simulink library "tqd"  (R2021b)
settings: Solver=VariableStepAuto  StartTime=0.0  StopTime=10.0  RelTol=1e-3
undefined symbols (not defined in the file or in its folder): ATQD_AccelLimitInRange_X_rpm, ATQD_AccelLimitInRange_Y_Nm, ATQD_AccelLimitOvrKi_X_Nm, ATQD_AccelLimitOvrKp_X_Nm, ATQD_BOSMapD_X_rpm, ATQD_BOSMapD_Y_pct, ATQD_BOSMapR_X_rpm, ATQD_BOSMapR_Y_pct, ATQD_HVBCurrSmooth_X_A, ATQD_LHMTqMapDLC_X_rpm, ATQD_LHMTqMapDLC_Y_pct, ATQD_LHMTqMapRLC_X_rpm, ATQD_LHMTqMapRLC_Y_pct, ATQD_NormalMapDLC_X_rpm, ATQD_NormalMapDLC_Y_pct, ATQD_NormalTqDecSR_X_rpm, ATQD_NormalTqDecSR_Y_Nm, ATQD_NormalTqIncSR_X_rpm, ATQD_NormalTqIncSR_Y_Nm, ATQD_OPDMapRLC_X_rpm, ATQD_OPDMapRLC_Y_pct, ATQD_RollRegTorReq_X_rpm, ATQD_RollRegTorReq_Y_enum, ATQD_VehSpdLimitInRange_X_rpm, ATQD_VehSpdLimitInRange_Y_Nm, ATQD_VehSpdLimitOvrKi_X_Nm, ATQD_VehSpdLimitOvrKp_X_Nm, EIGHT_INT, ENUM_BRAKEPEDAL_PRESSED, ENUM_BRAKEPEDAL_RELEASED, ENUM_COMBOKEY_DOWN, ENUM_COMBOKEY_M1, ENUM_COMBOKEY_M2, ENUM_COMBOKEY_NONE, ENUM_COMBOKEY_RKNEE, ENUM_COMBOKEY_STOPLV, ENUM_COMBOKEY_UP, ENUM_CP2VKNEEREQ_REQUEST, ENUM_CP2VNLVREQ_LEVEL1, ENUM_CP2VNLVREQ_LEVEL2, ENUM_CP2VNLVREQ_LOWER, ENUM_CP2VNLVREQ_STOPLV, ENUM_CP2VNLVREQ_UPPER, ENUM_CREEPIND_DISABLE, ENUM_CREEPIND_READY, ENUM_CREEPIND_RUNNING, ENUM_CREEPIND_WARNING, ENUM_DRIVELINERELEASE_RELEASE, ENUM_EBSTORQUERWQ_LIMIT, ENUM_EBSTORQUERWQ_TORQUE, ENUM_ECPVCUDRM_CONFORT, ENUM_ECPVCUDRM_ECO, ENUM_ECPVCUDRM_NORMAL, ENUM_ECPVCUDRM_NOTAVAILABLE, ENUM_EMTqModeDrvBrk_Accel, ENUM_EMTqModeDrvBrk_Brake, ENUM_EMTqModeDrvBrk_Coast, ENUM_ETC2ACTDRIVEDIR_BACKWARD, ENUM_ETC2ACTDRIVEDIR_FORWARD, ENUM_ETC2ACTDRIVEDIR_STILL ... (+341)
libraries: simulink x109, hcu_lib x67
(part 12 of 13)

== system tqd/TQD/Input_Convert/Input Signal Convert/Big Mike Combo V2 /Combo Key Detection/Function5/Key4 ==
  VTQD_ComboKeyCMD_enum : Inport
  VTQD_ComboKeyEn_flg : Inport  Port=2
  VTQD_ComboKeyReset_flg : Inport  Port=3
  VTQD_ComboKey3_enum : Inport  Port=4
  AND : Logic  Inputs=4  AllPortsSameDT=off  OutDataTypeStr=boolean
  Constant1 : Constant  Value=KTQD_Function5Off4_enum
  Constant2 : Constant  Value=ENUM_COMBOKEY_NONE
  Constant3 : Constant  Value=ENUM_COMBOKEY_NONE
  Constant4 : Constant  Value=ENUM_COMBOKEY_NONE
  Data Type Conversion : DataTypeConversion  OutDataTypeStr=uint8
  Delay : Delay  DelayLength=1  InitialCondition=uint8(0)
      settings: AttributesFormatString=%<InitialCondition>
  Delay1 : Delay  DelayLength=1  InitialCondition=uint8(0)
      settings: AttributesFormatString=%<InitialCondition>
  Delay2 : Delay  DelayLength=1  InitialCondition=uint8(0)
      settings: AttributesFormatString=%<InitialCondition>
  Detect Change : simulink/Logic and Bit Operations/Detect Change  vinit=boolean(0)  OutDataTypeStr=boolean
  Detect Increase : simulink/Logic and Bit Operations/Detect Increase  vinit=boolean(0)  OutDataTypeStr=boolean
  Equal : RelationalOperator  Operator===  OutDataTypeStr=boolean  RndMeth=Simplest
  Equal1 : RelationalOperator  Operator=~=  OutDataTypeStr=boolean  RndMeth=Simplest
  Equal2 : RelationalOperator  Operator=~=  OutDataTypeStr=boolean  RndMeth=Simplest
  Equal3 : RelationalOperator  Operator===  OutDataTypeStr=boolean  RndMeth=Simplest
  If : If  NumInputs=2  IfExpression=u1 ~=0  ElseIfExpressions=u2 ~= 0
  Maintain : Subsystem  TreatAsAtomicUnit=on
  Merge : Merge  Inputs=3
  OR : Logic  Operator=OR  AllPortsSameDT=off  OutDataTypeStr=boolean
  Reset : Subsystem  TreatAsAtomicUnit=on
  Write : Subsystem  TreatAsAtomicUnit=on
  VTQD_ComboKey4_enum : Outport
  VTQD_Key4Pass_flg : Outport  Port=2
  wires:
  [VTQD_ComboKey4_enum] -> Equal/1
  VTQD_ComboKeyEn_flg/1 -> [VTQD_ComboKeyEn_flg]
  VTQD_ComboKeyReset_flg/1 -> [VTQD_ComboKeyReset_flg]
  VTQD_ComboKeyCMD_enum/1 -> [VTQD_ComboKeyCMD_enum]
  Equal/1 -> [VTQD_Key4Pass_flg]  "VTQD_Function5Off4Pass_flg"
  Constant1/1 -> Equal/2
  If/2 -> Write/Action
  Write/1(WriteCMD) -> Merge/2
  If/1 -> Reset/Action
  Detect Increase/1 -> OR/1
  AND/1 -> [VTQD_WriteComboCMD_flg]  "VTQD_WriteComboCMD_flg"
  [VTQD_ComboKeyCMD_enum] -> Write/1(Input)
  [VTQD_ComboKeyCMD_enum] -> Detect Change/1
  [VTQD_ResetComboKey_flg] -> If/1
  [VTQD_ComboKeyEn_flg] -> Detect Increase/1
  Detect Change/1 -> AND/1
  Maintain/1(KeepKey4) -> Merge/3
  Constant4/1 -> Equal1/2
  If/3 -> Maintain/Action
  Delay/1 -> Equal2/1
  Merge/1 -> Data Type Conversion/1
  Reset/1(ResetToZero) -> Merge/1
  Equal2/1 -> AND/3
  Constant2/1 -> Equal2/2
  Equal1/1 -> AND/2
  [VTQD_ComboKey3_enum] -> Delay/1
  [VTQD_ComboKeyReset_flg] -> OR/2
  [VTQD_ComboKeyCMD_enum] -> Equal1/1
  [VTQD_WriteComboCMD_flg] -> If/2
  OR/1 -> [VTQD_ResetComboKey_flg]  "VTQD_ResetComboKey_flg"
  VTQD_ComboKey3_enum/1 -> [VTQD_ComboKey3_enum]
  [VTQD_ComboKey4_enum] -> Delay1/1
  Constant3/1 -> Equal3/2
  Delay1/1 -> Equal3/1
  Equal3/1 -> AND/4
  [VTQD_Key4Pass_flg] -> VTQD_Key4Pass_flg/1
  [VTQD_ComboKey4_enum] -> VTQD_ComboKey4_enum/1
  [VTQD_ComboKey4_enum] -> Delay2/1
  Delay2/1 -> Maintain/1(Input)
  Data Type Conversion/1 -> [VTQD_ComboKey4_enum]  "VTQD_Function5Off4_enum"

== system tqd/TQD/Input_Convert/Input Signal Convert/Big Mike Combo V2 /Combo Key Detection/Function5/Key5 ==
  VTQD_ComboKeyCMD_enum : Inport
  VTQD_ComboKeyEn_flg : Inport  Port=2
  VTQD_ComboKeyReset_flg : Inport  Port=3
  VTQD_ComboKey4_enum : Inport  Port=4
  AND : Logic  Inputs=4  AllPortsSameDT=off  OutDataTypeStr=boolean
  Constant1 : Constant  Value=KTQD_Function5Off5_enum
  Constant2 : Constant  Value=ENUM_COMBOKEY_NONE
  Constant3 : Constant  Value=ENUM_COMBOKEY_NONE
  Constant4 : Constant  Value=ENUM_COMBOKEY_NONE
  Data Type Conversion : DataTypeConversion  OutDataTypeStr=uint8
  Delay : Delay  DelayLength=1  InitialCondition=uint8(0)
      settings: AttributesFormatString=%<InitialCondition>
  Delay1 : Delay  DelayLength=1  InitialCondition=uint8(0)
      settings: AttributesFormatString=%<InitialCondition>
  Delay2 : Delay  DelayLength=1  InitialCondition=uint8(0)
      settings: AttributesFormatString=%<InitialCondition>
  Detect Change : simulink/Logic and Bit Operations/Detect Change  vinit=boolean(0)  OutDataTypeStr=boolean
  Detect Increase : simulink/Logic and Bit Operations/Detect Increase  vinit=boolean(0)  OutDataTypeStr=boolean
  Equal : RelationalOperator  Operator===  OutDataTypeStr=boolean  RndMeth=Simplest
  Equal1 : RelationalOperator  Operator=~=  OutDataTypeStr=boolean  RndMeth=Simplest
  Equal2 : RelationalOperator  Operator=~=  OutDataTypeStr=boolean  RndMeth=Simplest
  Equal3 : RelationalOperator  Operator===  OutDataTypeStr=boolean  RndMeth=Simplest
  If : If  NumInputs=2  IfExpression=u1 ~=0  ElseIfExpressions=u2 ~= 0
  Maintain : Subsystem  TreatAsAtomicUnit=on
  Merge : Merge  Inputs=3
  OR : Logic  Operator=OR  AllPortsSameDT=off  OutDataTypeStr=boolean
  Reset : Subsystem  TreatAsAtomicUnit=on
  Write : Subsystem  TreatAsAtomicUnit=on
  VTQD_ComboKey5_enum : Outport
  VTQD_Key5Pass_flg : Outport  Port=2
  wires:
  [VTQD_Key5Pass_flg] -> VTQD_Key5Pass_flg/1
  Equal3/1 -> AND/4
  Delay1/1 -> Equal3/1
  Constant3/1 -> Equal3/2
  [VTQD_ComboKey5_enum] -> Delay1/1
  VTQD_ComboKey4_enum/1 -> [VTQD_ComboKey4_enum]
  OR/1 -> [VTQD_ResetComboKey_flg]  "VTQD_ResetComboKey_flg"
  [VTQD_WriteComboCMD_flg] -> If/2
  [VTQD_ComboKeyCMD_enum] -> Equal1/1
  [VTQD_ComboKeyReset_flg] -> OR/2
  [VTQD_ComboKey4_enum] -> Delay/1
  Equal1/1 -> AND/2
  Constant2/1 -> Equal2/2
  Equal2/1 -> AND/3
  Reset/1(ResetToZero) -> Merge/1
  Merge/1 -> Data Type Conversion/1
  Delay/1 -> Equal2/1
  If/3 -> Maintain/Action
  Constant4/1 -> Equal1/2
  Maintain/1(KeepKey5) -> Merge/3
  Detect Change/1 -> AND/1
  [VTQD_ComboKeyEn_flg] -> Detect Increase/1
  [VTQD_ResetComboKey_flg] -> If/1
  [VTQD_ComboKeyCMD_enum] -> Detect Change/1
  [VTQD_ComboKeyCMD_enum] -> Write/1(Input)
  AND/1 -> [VTQD_WriteComboCMD_flg]  "VTQD_WriteComboCMD_flg"
  Detect Increase/1 -> OR/1
  If/1 -> Reset/Action
  Write/1(WriteCMD) -> Merge/2
  If/2 -> Write/Action
  Constant1/1 -> Equal/2
  Equal/1 -> [VTQD_Key5Pass_flg]  "VTQD_Function5Off5Pass_flg"
  VTQD_ComboKeyCMD_enum/1 -> [VTQD_ComboKeyCMD_enum]
  VTQD_ComboKeyReset_flg/1 -> [VTQD_ComboKeyReset_flg]
  VTQD_ComboKeyEn_flg/1 -> [VTQD_ComboKeyEn_flg]
  [VTQD_ComboKey5_enum] -> Equal/1
  [VTQD_ComboKey5_enum] -> VTQD_ComboKey5_enum/1
  [VTQD_ComboKey5_enum] -> Delay2/1
  Delay2/1 -> Maintain/1(Input)
  Data Type Conversion/1 -> [VTQD_ComboKey5_enum]  "VTQD_Function5Off5_enum"

== system tqd/TQD/Input_Convert/Input Signal Convert/Big Mike Combo V2 /Combo Key Detection/Function5/Key6 ==
  VTQD_ComboKeyCMD_enum : Inport
  VTQD_ComboKeyEn_flg : Inport  Port=2
  VTQD_ComboKeyReset_flg : Inport  Port=3
  VTQD_ComboKey5_enum : Inport  Port=4
  AND : Logic  Inputs=4  AllPortsSameDT=off  OutDataTypeStr=boolean
  Constant1 : Constant  Value=KTQD_Function5Off6_enum
  Constant2 : Constant  Value=ENUM_COMBOKEY_NONE
  Constant3 : Constant  Value=ENUM_COMBOKEY_NONE
  Constant4 : Constant  Value=ENUM_COMBOKEY_NONE
  Data Type Conversion : DataTypeConversion  OutDataTypeStr=uint8
  Delay : Delay  DelayLength=1  InitialCondition=uint8(0)
      settings: AttributesFormatString=%<InitialCondition>
  Delay1 : Delay  DelayLength=1  InitialCondition=uint8(0)
      settings: AttributesFormatString=%<InitialCondition>
  Delay2 : Delay  DelayLength=1  InitialCondition=uint8(0)
      settings: AttributesFormatString=%<InitialCondition>
  Detect Change : simulink/Logic and Bit Operations/Detect Change  vinit=boolean(0)  OutDataTypeStr=boolean
  Detect Increase : simulink/Logic and Bit Operations/Detect Increase  vinit=boolean(0)  OutDataTypeStr=boolean
  Equal : RelationalOperator  Operator===  OutDataTypeStr=boolean  RndMeth=Simplest
  Equal1 : RelationalOperator  Operator=~=  OutDataTypeStr=boolean  RndMeth=Simplest
  Equal2 : RelationalOperator  Operator=~=  OutDataTypeStr=boolean  RndMeth=Simplest
  Equal3 : RelationalOperator  Operator===  OutDataTypeStr=boolean  RndMeth=Simplest
  If : If  NumInputs=2  IfExpression=u1 ~=0  ElseIfExpressions=u2 ~= 0
  Maintain : Subsystem  TreatAsAtomicUnit=on
  Merge : Merge  Inputs=3
  OR : Logic  Operator=OR  AllPortsSameDT=off  OutDataTypeStr=boolean
  Reset : Subsystem  TreatAsAtomicUnit=on
  Write : Subsystem  TreatAsAtomicUnit=on
  VTQD_ComboKey6_enum : Outport
  VTQD_Key6Pass_flg : Outport  Port=2
  wires:
  [VTQD_ComboKey6_enum] -> VTQD_ComboKey6_enum/1
  [VTQD_ComboKey6_enum] -> Equal/1
  VTQD_ComboKeyEn_flg/1 -> [VTQD_ComboKeyEn_flg]
  VTQD_ComboKeyReset_flg/1 -> [VTQD_ComboKeyReset_flg]
  VTQD_ComboKeyCMD_enum/1 -> [VTQD_ComboKeyCMD_enum]
  Equal/1 -> [VTQD_Key6Pass_flg]  "VTQD_Function5Off6Pass_flg"
  Constant1/1 -> Equal/2
  If/2 -> Write/Action
  Write/1(WriteCMD) -> Merge/2
  If/1 -> Reset/Action
  Detect Increase/1 -> OR/1
  AND/1 -> [VTQD_WriteComboCMD_flg]  "VTQD_WriteComboCMD_flg"
  [VTQD_ComboKeyCMD_enum] -> Write/1(Input)
  [VTQD_ComboKeyCMD_enum] -> Detect Change/1
  [VTQD_ResetComboKey_flg] -> If/1
  [VTQD_ComboKeyEn_flg] -> Detect Increase/1
  Detect Change/1 -> AND/1
  Maintain/1(KeepKey6) -> Merge/3
  Constant4/1 -> Equal1/2
  If/3 -> Maintain/Action
  Delay/1 -> Equal2/1
  Merge/1 -> Data Type Conversion/1
  Reset/1(ResetToZero) -> Merge/1
  Equal2/1 -> AND/3
  Constant2/1 -> Equal2/2
  Equal1/1 -> AND/2
  [VTQD_ComboKey5_enum] -> Delay/1
  [VTQD_ComboKeyReset_flg] -> OR/2
  [VTQD_ComboKeyCMD_enum] -> Equal1/1
  [VTQD_WriteComboCMD_flg] -> If/2
  OR/1 -> [VTQD_ResetComboKey_flg]  "VTQD_ResetComboKey_flg"
  VTQD_ComboKey5_enum/1 -> [VTQD_ComboKey5_enum]
  [VTQD_ComboKey6_enum] -> Delay1/1
  Constant3/1 -> Equal3/2
  Delay1/1 -> Equal3/1
  Equal3/1 -> AND/4
  [VTQD_Key6Pass_flg] -> VTQD_Key6Pass_flg/1
  Delay2/1 -> Maintain/1(Input)
  [VTQD_ComboKey6_enum] -> Delay2/1
  Data Type Conversion/1 -> [VTQD_ComboKey6_enum]  "VTQD_Function5Off6_enum"

== system tqd/TQD/Input_Convert/Input Signal Convert/Big Mike Combo V2 /Combo Key Detection/Function5/Key7 ==
  VTQD_ComboKeyCMD_enum : Inport
  VTQD_ComboKeyEn_flg : Inport  Port=2
  VTQD_ComboKeyReset_flg : Inport  Port=3
  VTQD_ComboKey6_enum : Inport  Port=4
  AND : Logic  Inputs=4  AllPortsSameDT=off  OutDataTypeStr=boolean
  Constant1 : Constant  Value=KTQD_Function5Off7_enum
  Constant2 : Constant  Value=ENUM_COMBOKEY_NONE  OutDataTypeStr=uint8
  Constant3 : Constant  Value=ENUM_COMBOKEY_NONE
  Constant4 : Constant  Value=ENUM_COMBOKEY_NONE  OutDataTypeStr=uint8
  Data Type Conversion : DataTypeConversion  OutDataTypeStr=uint8
  Delay : Delay  DelayLength=1  InitialCondition=uint8(0)
      settings: AttributesFormatString=%<InitialCondition>
  Delay1 : Delay  DelayLength=1  InitialCondition=uint8(0)
      settings: AttributesFormatString=%<InitialCondition>
  Delay2 : Delay  DelayLength=1  InitialCondition=uint8(0)
      settings: AttributesFormatString=%<InitialCondition>
  Detect Change : simulink/Logic and Bit Operations/Detect Change  vinit=boolean(0)  OutDataTypeStr=boolean
  Detect Increase : simulink/Logic and Bit Operations/Detect Increase  vinit=boolean(0)  OutDataTypeStr=boolean
  Equal : RelationalOperator  Operator===  OutDataTypeStr=boolean  RndMeth=Simplest
  Equal1 : RelationalOperator  Operator=~=  OutDataTypeStr=boolean  RndMeth=Simplest
  Equal2 : RelationalOperator  Operator=~=  OutDataTypeStr=boolean  RndMeth=Simplest
  Equal3 : RelationalOperator  Operator===  OutDataTypeStr=boolean  RndMeth=Simplest
  If : If  NumInputs=2  IfExpression=u1 ~=0  ElseIfExpressions=u2 ~= 0
  Maintain : Subsystem  TreatAsAtomicUnit=on
  Merge : Merge  Inputs=3
  OR : Logic  Operator=OR  AllPortsSameDT=off  OutDataTypeStr=boolean
  Reset : Subsystem  TreatAsAtomicUnit=on
  Write : Subsystem  TreatAsAtomicUnit=on
  VTQD_ComboKey7_enum : Outport
  VTQD_Key7Pass_flg : Outport  Port=2
  wires:
  [VTQD_Key7Pass_flg] -> VTQD_Key7Pass_flg/1
  Equal3/1 -> AND/4
  Delay1/1 -> Equal3/1
  Constant3/1 -> Equal3/2
  [VTQD_ComboKey7_enum] -> Delay1/1
  VTQD_ComboKey6_enum/1 -> [VTQD_ComboKey6_enum]
  OR/1 -> [VTQD_ResetComboKey_flg]  "VTQD_ResetComboKey_flg"
  [VTQD_WriteComboCMD_flg] -> If/2
  [VTQD_ComboKeyCMD_enum] -> Equal1/1
  [VTQD_ComboKeyReset_flg] -> OR/2
  [VTQD_ComboKey6_enum] -> Delay/1
  Equal1/1 -> AND/2
  Constant2/1 -> Equal2/2
  Equal2/1 -> AND/3
  Reset/1(ResetToZero) -> Merge/1
  Merge/1 -> Data Type Conversion/1
  Delay/1 -> Equal2/1
  If/3 -> Maintain/Action
  Constant4/1 -> Equal1/2
  Maintain/1(KeepKey7) -> Merge/3
  Detect Change/1 -> AND/1
  [VTQD_ComboKeyEn_flg] -> Detect Increase/1
  [VTQD_ResetComboKey_flg] -> If/1
  [VTQD_ComboKeyCMD_enum] -> Detect Change/1
  [VTQD_ComboKeyCMD_enum] -> Write/1(Input)
  AND/1 -> [VTQD_WriteComboCMD_flg]  "VTQD_WriteComboCMD_flg"
  Detect Increase/1 -> OR/1
  If/1 -> Reset/Action
  Write/1(WriteCMD) -> Merge/2
  If/2 -> Write/Action
  Constant1/1 -> Equal/2
  Equal/1 -> [VTQD_Key7Pass_flg]  "VTQD_Function5Off7Pass_flg"
  VTQD_ComboKeyCMD_enum/1 -> [VTQD_ComboKeyCMD_enum]
  VTQD_ComboKeyReset_flg/1 -> [VTQD_ComboKeyReset_flg]
  VTQD_ComboKeyEn_flg/1 -> [VTQD_ComboKeyEn_flg]
  [VTQD_ComboKey7_enum] -> Equal/1
  [VTQD_ComboKey7_enum] -> VTQD_ComboKey7_enum/1
  [VTQD_ComboKey7_enum] -> Delay2/1
  Delay2/1 -> Maintain/1(Input)
  Data Type Conversion/1 -> [VTQD_ComboKey7_enum]  "VTQD_Function5Off7_enum"

== system tqd/TQD/Input_Convert/Input Signal Convert/Big Mike Combo V2 /Combo Key Detection/Function5/Key8 ==
  VTQD_ComboKeyCMD_enum : Inport
  VTQD_ComboKeyEn_flg : Inport  Port=2
  VTQD_ComboKeyReset_flg : Inport  Port=3
  VTQD_ComboKey7_enum : Inport  Port=4
  AND : Logic  Inputs=4  AllPortsSameDT=off  OutDataTypeStr=boolean
  Constant1 : Constant  Value=KTQD_Function5Off8_enum
  Constant2 : Constant  Value=ENUM_COMBOKEY_NONE
  Constant3 : Constant  Value=ENUM_COMBOKEY_NONE
  Constant4 : Constant  Value=ENUM_COMBOKEY_NONE
  Data Type Conversion : DataTypeConversion  OutDataTypeStr=uint8
  Delay : Delay  DelayLength=1  InitialCondition=uint8(0)
      settings: AttributesFormatString=%<InitialCondition>
  Delay1 : Delay  DelayLength=1  InitialCondition=uint8(0)
      settings: AttributesFormatString=%<InitialCondition>
  Delay2 : Delay  DelayLength=1  InitialCondition=uint8(0)
      settings: AttributesFormatString=%<InitialCondition>
  Detect Change : simulink/Logic and Bit Operations/Detect Change  vinit=boolean(0)  OutDataTypeStr=boolean
  Detect Increase : simulink/Logic and Bit Operations/Detect Increase  vinit=boolean(0)  OutDataTypeStr=boolean
  Equal : RelationalOperator  Operator===  OutDataTypeStr=boolean  RndMeth=Simplest
  Equal1 : RelationalOperator  Operator=~=  OutDataTypeStr=boolean  RndMeth=Simplest
  Equal2 : RelationalOperator  Operator=~=  OutDataTypeStr=boolean  RndMeth=Simplest
  Equal3 : RelationalOperator  Operator===  OutDataTypeStr=boolean  RndMeth=Simplest
  If : If  NumInputs=2  IfExpression=u1 ~=0  ElseIfExpressions=u2 ~= 0
  Maintain : Subsystem  TreatAsAtomicUnit=on
  Merge : Merge  Inputs=3
  OR : Logic  Operator=OR  AllPortsSameDT=off  OutDataTypeStr=boolean
  Reset : Subsystem  TreatAsAtomicUnit=on
  Write : Subsystem  TreatAsAtomicUnit=on
  VTQD_ComboKey8_enum : Outport
  VTQD_Key8Pass_flg : Outport  Port=2
  wires:
  VTQD_ComboKeyEn_flg/1 -> [VTQD_ComboKeyEn_flg]
  VTQD_ComboKeyReset_flg/1 -> [VTQD_ComboKeyReset_flg]
  VTQD_ComboKeyCMD_enum/1 -> [VTQD_ComboKeyCMD_enum]
  Equal/1 -> [VTQD_Key8Pass_flg]  "VTQD_Function5Off8Pass_flg"
  Constant1/1 -> Equal/2
  If/2 -> Write/Action
  Write/1(WriteCMD) -> Merge/2
  If/1 -> Reset/Action
  Detect Increase/1 -> OR/1
  AND/1 -> [VTQD_WriteComboCMD_flg]  "VTQD_WriteComboCMD_flg"
  [VTQD_ComboKeyCMD_enum] -> Write/1(Input)
  [VTQD_ComboKeyCMD_enum] -> Detect Change/1
  [VTQD_ResetComboKey_flg] -> If/1
  [VTQD_ComboKeyEn_flg] -> Detect Increase/1
  Detect Change/1 -> AND/1
  Maintain/1(KeepKey8) -> Merge/3
  Constant4/1 -> Equal1/2
  If/3 -> Maintain/Action
  Delay/1 -> Equal2/1
  Merge/1 -> Data Type Conversion/1
  Reset/1(ResetToZero) -> Merge/1
  Equal2/1 -> AND/3
  Constant2/1 -> Equal2/2
  Equal1/1 -> AND/2
  [VTQD_ComboKey7_enum] -> Delay/1
  [VTQD_ComboKeyReset_flg] -> OR/2
  [VTQD_ComboKeyCMD_enum] -> Equal1/1
  [VTQD_WriteComboCMD_flg] -> If/2
  OR/1 -> [VTQD_ResetComboKey_flg]  "VTQD_ResetComboKey_flg"
  VTQD_ComboKey7_enum/1 -> [VTQD_ComboKey7_enum]
  [VTQD_ComboKey8_enum] -> Delay1/1
  Constant3/1 -> Equal3/2
  Delay1/1 -> Equal3/1
  Equal3/1 -> AND/4
  [VTQD_Key8Pass_flg] -> VTQD_Key8Pass_flg/1
  [VTQD_ComboKey8_enum] -> Equal/1
  [VTQD_ComboKey8_enum] -> VTQD_ComboKey8_enum/1
  [VTQD_ComboKey8_enum] -> Delay2/1
  Delay2/1 -> Maintain/1(Input)
  Data Type Conversion/1 -> [VTQD_ComboKey8_enum]  "VTQD_Function5Off8_enum"

== system tqd/TQD/Input_Convert/Input Signal Convert/Big Mike Combo V2 /Combo Key Detection/Function1 Alcohol Lock/Key1/Maintain ==
  Input : Inport
  Action Port : ActionPort
  KeepKey1 : Outport
  wires:
  Input/1 -> KeepKey1/1

== system tqd/TQD/Input_Convert/Input Signal Convert/Big Mike Combo V2 /Combo Key Detection/Function1 Alcohol Lock/Key1/Reset ==
  Action Port : ActionPort
  Constant : Constant  Value=ENUM_COMBOKEY_NONE
  ResetToZero : Outport
  wires:
  Constant/1 -> ResetToZero/1

== system tqd/TQD/Input_Convert/Input Signal Convert/Big Mike Combo V2 /Combo Key Detection/Function1 Alcohol Lock/Key1/Write ==
  Input : Inport
  Action Port : ActionPort
  WriteCMD : Outport
  wires:
  Input/1 -> WriteCMD/1

== system tqd/TQD/Input_Convert/Input Signal Convert/Big Mike Combo V2 /Combo Key Detection/Function1 Alcohol Lock/Key2/Maintain ==
  Input : Inport
  Action Port : ActionPort
  KeepKey2 : Outport
  wires:
  Input/1 -> KeepKey2/1

== system tqd/TQD/Input_Convert/Input Signal Convert/Big Mike Combo V2 /Combo Key Detection/Function1 Alcohol Lock/Key2/Reset ==
  Action Port : ActionPort
  Constant : Constant  Value=ENUM_COMBOKEY_NONE
  ResetToZero : Outport
  wires:
  Constant/1 -> ResetToZero/1

== system tqd/TQD/Input_Convert/Input Signal Convert/Big Mike Combo V2 /Combo Key Detection/Function1 Alcohol Lock/Key2/Write ==
  Input : Inport
  Action Port : ActionPort
  WriteCMD : Outport
  wires:
  Input/1 -> WriteCMD/1

== system tqd/TQD/Input_Convert/Input Signal Convert/Big Mike Combo V2 /Combo Key Detection/Function1 Alcohol Lock/Key3/Maintain ==
  Input : Inport
  Action Port : ActionPort
  KeepKey3 : Outport
  wires:
  Input/1 -> KeepKey3/1

== system tqd/TQD/Input_Convert/Input Signal Convert/Big Mike Combo V2 /Combo Key Detection/Function1 Alcohol Lock/Key3/Reset ==
  Action Port : ActionPort
  Constant : Constant  Value=ENUM_COMBOKEY_NONE
  ResetToZero : Outport
  wires:
  Constant/1 -> ResetToZero/1

== system tqd/TQD/Input_Convert/Input Signal Convert/Big Mike Combo V2 /Combo Key Detection/Function1 Alcohol Lock/Key3/Write ==
  Input : Inport
  Action Port : ActionPort
  WriteCMD : Outport
  wires:
  Input/1 -> WriteCMD/1

== system tqd/TQD/Input_Convert/Input Signal Convert/Big Mike Combo V2 /Combo Key Detection/Function1 Alcohol Lock/Key4/Maintain ==
  Input : Inport
  Action Port : ActionPort
  KeepKey4 : Outport
  wires:
  Input/1 -> KeepKey4/1

== system tqd/TQD/Input_Convert/Input Signal Convert/Big Mike Combo V2 /Combo Key Detection/Function1 Alcohol Lock/Key4/Reset ==
  Action Port : ActionPort
  Constant : Constant  Value=ENUM_COMBOKEY_NONE
  ResetToZero : Outport
  wires:
  Constant/1 -> ResetToZero/1

== system tqd/TQD/Input_Convert/Input Signal Convert/Big Mike Combo V2 /Combo Key Detection/Function1 Alcohol Lock/Key4/Write ==
  Input : Inport
  Action Port : ActionPort
  WriteCMD : Outport
  wires:
  Input/1 -> WriteCMD/1

== system tqd/TQD/Input_Convert/Input Signal Convert/Big Mike Combo V2 /Combo Key Detection/Function1 Alcohol Lock/Key5/Maintain ==
  Input : Inport
  Action Port : ActionPort
  KeepKey5 : Outport
  wires:
  Input/1 -> KeepKey5/1

== system tqd/TQD/Input_Convert/Input Signal Convert/Big Mike Combo V2 /Combo Key Detection/Function1 Alcohol Lock/Key5/Reset ==
  Action Port : ActionPort
  Constant : Constant  Value=ENUM_COMBOKEY_NONE
  ResetToZero : Outport
  wires:
  Constant/1 -> ResetToZero/1

== system tqd/TQD/Input_Convert/Input Signal Convert/Big Mike Combo V2 /Combo Key Detection/Function1 Alcohol Lock/Key5/Write ==
  Input : Inport
  Action Port : ActionPort
  WriteCMD : Outport
  wires:
  Input/1 -> WriteCMD/1

== system tqd/TQD/Input_Convert/Input Signal Convert/Big Mike Combo V2 /Combo Key Detection/Function1 Alcohol Lock/Key6/Maintain ==
  Input : Inport
  Action Port : ActionPort
  KeepKey6 : Outport
  wires:
  Input/1 -> KeepKey6/1

== system tqd/TQD/Input_Convert/Input Signal Convert/Big Mike Combo V2 /Combo Key Detection/Function1 Alcohol Lock/Key6/Reset ==
  Action Port : ActionPort
  Constant : Constant  Value=ENUM_COMBOKEY_NONE
  ResetToZero : Outport
  wires:
  Constant/1 -> ResetToZero/1

== system tqd/TQD/Input_Convert/Input Signal Convert/Big Mike Combo V2 /Combo Key Detection/Function1 Alcohol Lock/Key6/Write ==
  Input : Inport
  Action Port : ActionPort
  WriteCMD : Outport
  wires:
  Input/1 -> WriteCMD/1

== system tqd/TQD/Input_Convert/Input Signal Convert/Big Mike Combo V2 /Combo Key Detection/Function1 Alcohol Lock/Key7/Maintain ==
  Input : Inport
  Action Port : ActionPort
  KeepKey7 : Outport
  wires:
  Input/1 -> KeepKey7/1

== system tqd/TQD/Input_Convert/Input Signal Convert/Big Mike Combo V2 /Combo Key Detection/Function1 Alcohol Lock/Key7/Reset ==
  Action Port : ActionPort
  Constant : Constant  Value=ENUM_COMBOKEY_NONE
  ResetToZero : Outport
  wires:
  Constant/1 -> ResetToZero/1

== system tqd/TQD/Input_Convert/Input Signal Convert/Big Mike Combo V2 /Combo Key Detection/Function1 Alcohol Lock/Key7/Write ==
  Input : Inport
  Action Port : ActionPort
  WriteCMD : Outport
  wires:
  Input/1 -> WriteCMD/1

== system tqd/TQD/Input_Convert/Input Signal Convert/Big Mike Combo V2 /Combo Key Detection/Function1 Alcohol Lock/Key8/Maintain ==
  Input : Inport
  Action Port : ActionPort
  KeepKey8 : Outport
  wires:
  Input/1 -> KeepKey8/1

== system tqd/TQD/Input_Convert/Input Signal Convert/Big Mike Combo V2 /Combo Key Detection/Function1 Alcohol Lock/Key8/Reset ==
  Action Port : ActionPort
  Constant : Constant  Value=ENUM_COMBOKEY_NONE
  ResetToZero : Outport
  wires:
  Constant/1 -> ResetToZero/1

== system tqd/TQD/Input_Convert/Input Signal Convert/Big Mike Combo V2 /Combo Key Detection/Function1 Alcohol Lock/Key8/Write ==
  Input : Inport
  Action Port : ActionPort
  WriteCMD : Outport
  wires:
  Input/1 -> WriteCMD/1

== system tqd/TQD/Input_Convert/Input Signal Convert/Big Mike Combo V2 /Combo Key Detection/Function2 /Key1/Maintain ==
  Input : Inport
  Action Port : ActionPort
  KeepKey1 : Outport
  wires:
  Input/1 -> KeepKey1/1

== system tqd/TQD/Input_Convert/Input Signal Convert/Big Mike Combo V2 /Combo Key Detection/Function2 /Key1/Reset ==
  Action Port : ActionPort
  Constant : Constant  Value=ENUM_COMBOKEY_NONE
  ResetToZero : Outport
  wires:
  Constant/1 -> ResetToZero/1

== system tqd/TQD/Input_Convert/Input Signal Convert/Big Mike Combo V2 /Combo Key Detection/Function2 /Key1/Write ==
  Input : Inport
  Action Port : ActionPort
  WriteCMD : Outport
  wires:
  Input/1 -> WriteCMD/1

== system tqd/TQD/Input_Convert/Input Signal Convert/Big Mike Combo V2 /Combo Key Detection/Function2 /Key2/Maintain ==
  Input : Inport
  Action Port : ActionPort
  KeepKey2 : Outport
  wires:
  Input/1 -> KeepKey2/1

== system tqd/TQD/Input_Convert/Input Signal Convert/Big Mike Combo V2 /Combo Key Detection/Function2 /Key2/Reset ==
  Action Port : ActionPort
  Constant : Constant  Value=ENUM_COMBOKEY_NONE
  ResetToZero : Outport
  wires:
  Constant/1 -> ResetToZero/1

== system tqd/TQD/Input_Convert/Input Signal Convert/Big Mike Combo V2 /Combo Key Detection/Function2 /Key2/Write ==
  Input : Inport
  Action Port : ActionPort
  WriteCMD : Outport
  wires:
  Input/1 -> WriteCMD/1

== system tqd/TQD/Input_Convert/Input Signal Convert/Big Mike Combo V2 /Combo Key Detection/Function2 /Key3/Maintain ==
  Input : Inport
  Action Port : ActionPort
  KeepKey3 : Outport
  wires:
  Input/1 -> KeepKey3/1

== system tqd/TQD/Input_Convert/Input Signal Convert/Big Mike Combo V2 /Combo Key Detection/Function2 /Key3/Reset ==
  Action Port : ActionPort
  Constant : Constant  Value=ENUM_COMBOKEY_NONE
  ResetToZero : Outport
  wires:
  Constant/1 -> ResetToZero/1

== system tqd/TQD/Input_Convert/Input Signal Convert/Big Mike Combo V2 /Combo Key Detection/Function2 /Key3/Write ==
  Input : Inport
  Action Port : ActionPort
  WriteCMD : Outport
  wires:
  Input/1 -> WriteCMD/1

== system tqd/TQD/Input_Convert/Input Signal Convert/Big Mike Combo V2 /Combo Key Detection/Function2 /Key4/Maintain ==
  Input : Inport
  Action Port : ActionPort
  KeepKey4 : Outport
  wires:
  Input/1 -> KeepKey4/1

== system tqd/TQD/Input_Convert/Input Signal Convert/Big Mike Combo V2 /Combo Key Detection/Function2 /Key4/Reset ==
  Action Port : ActionPort
  Constant : Constant  Value=ENUM_COMBOKEY_NONE
  ResetToZero : Outport
  wires:
  Constant/1 -> ResetToZero/1

== system tqd/TQD/Input_Convert/Input Signal Convert/Big Mike Combo V2 /Combo Key Detection/Function2 /Key4/Write ==
  Input : Inport
  Action Port : ActionPort
  WriteCMD : Outport
  wires:
  Input/1 -> WriteCMD/1

== system tqd/TQD/Input_Convert/Input Signal Convert/Big Mike Combo V2 /Combo Key Detection/Function2 /Key5/Maintain ==
  Input : Inport
  Action Port : ActionPort
  KeepKey5 : Outport
  wires:
  Input/1 -> KeepKey5/1

== system tqd/TQD/Input_Convert/Input Signal Convert/Big Mike Combo V2 /Combo Key Detection/Function2 /Key5/Reset ==
  Action Port : ActionPort
  Constant : Constant  Value=ENUM_COMBOKEY_NONE
  ResetToZero : Outport
  wires:
  Constant/1 -> ResetToZero/1

== system tqd/TQD/Input_Convert/Input Signal Convert/Big Mike Combo V2 /Combo Key Detection/Function2 /Key5/Write ==
  Input : Inport
  Action Port : ActionPort
  WriteCMD : Outport
  wires:
  Input/1 -> WriteCMD/1

== system tqd/TQD/Input_Convert/Input Signal Convert/Big Mike Combo V2 /Combo Key Detection/Function2 /Key6/Maintain ==
  Input : Inport
  Action Port : ActionPort
  KeepKey6 : Outport
  wires:
  Input/1 -> KeepKey6/1

== system tqd/TQD/Input_Convert/Input Signal Convert/Big Mike Combo V2 /Combo Key Detection/Function2 /Key6/Reset ==
  Action Port : ActionPort
  Constant : Constant  Value=ENUM_COMBOKEY_NONE
  ResetToZero : Outport
  wires:
  Constant/1 -> ResetToZero/1

== system tqd/TQD/Input_Convert/Input Signal Convert/Big Mike Combo V2 /Combo Key Detection/Function2 /Key6/Write ==
  Input : Inport
  Action Port : ActionPort
  WriteCMD : Outport
  wires:
  Input/1 -> WriteCMD/1

== system tqd/TQD/Input_Convert/Input Signal Convert/Big Mike Combo V2 /Combo Key Detection/Function2 /Key7/Maintain ==
  Input : Inport
  Action Port : ActionPort
  KeepKey7 : Outport
  wires:
  Input/1 -> KeepKey7/1

== system tqd/TQD/Input_Convert/Input Signal Convert/Big Mike Combo V2 /Combo Key Detection/Function2 /Key7/Reset ==
  Action Port : ActionPort
  Constant : Constant  Value=ENUM_COMBOKEY_NONE
  ResetToZero : Outport
  wires:
  Constant/1 -> ResetToZero/1

== system tqd/TQD/Input_Convert/Input Signal Convert/Big Mike Combo V2 /Combo Key Detection/Function2 /Key7/Write ==
  Input : Inport
  Action Port : ActionPort
  WriteCMD : Outport
  wires:
  Input/1 -> WriteCMD/1

== system tqd/TQD/Input_Convert/Input Signal Convert/Big Mike Combo V2 /Combo Key Detection/Function2 /Key8/Maintain ==
  Input : Inport
  Action Port : ActionPort
  KeepKey8 : Outport
  wires:
  Input/1 -> KeepKey8/1

== system tqd/TQD/Input_Convert/Input Signal Convert/Big Mike Combo V2 /Combo Key Detection/Function2 /Key8/Reset ==
  Action Port : ActionPort
  Constant : Constant  Value=ENUM_COMBOKEY_NONE
  ResetToZero : Outport
  wires:
  Constant/1 -> ResetToZero/1

== system tqd/TQD/Input_Convert/Input Signal Convert/Big Mike Combo V2 /Combo Key Detection/Function2 /Key8/Write ==
  Input : Inport
  Action Port : ActionPort
  WriteCMD : Outport
  wires:
  Input/1 -> WriteCMD/1

== system tqd/TQD/Input_Convert/Input Signal Convert/Big Mike Combo V2 /Combo Key Detection/Function3/Key1/Maintain ==
  Input : Inport
  Action Port : ActionPort
  KeepKey1 : Outport
  wires:
  Input/1 -> KeepKey1/1

== system tqd/TQD/Input_Convert/Input Signal Convert/Big Mike Combo V2 /Combo Key Detection/Function3/Key1/Reset ==
  Action Port : ActionPort
  Constant : Constant  Value=ENUM_COMBOKEY_NONE
  ResetToZero : Outport
  wires:
  Constant/1 -> ResetToZero/1

== system tqd/TQD/Input_Convert/Input Signal Convert/Big Mike Combo V2 /Combo Key Detection/Function3/Key1/Write ==
  Input : Inport
  Action Port : ActionPort
  WriteCMD : Outport
  wires:
  Input/1 -> WriteCMD/1

== system tqd/TQD/Input_Convert/Input Signal Convert/Big Mike Combo V2 /Combo Key Detection/Function3/Key2/Maintain ==
  Input : Inport
  Action Port : ActionPort
  KeepKey2 : Outport
  wires:
  Input/1 -> KeepKey2/1

== system tqd/TQD/Input_Convert/Input Signal Convert/Big Mike Combo V2 /Combo Key Detection/Function3/Key2/Reset ==
  Action Port : ActionPort
  Constant : Constant  Value=ENUM_COMBOKEY_NONE
  ResetToZero : Outport
  wires:
  Constant/1 -> ResetToZero/1

== system tqd/TQD/Input_Convert/Input Signal Convert/Big Mike Combo V2 /Combo Key Detection/Function3/Key2/Write ==
  Input : Inport
  Action Port : ActionPort
  WriteCMD : Outport
  wires:
  Input/1 -> WriteCMD/1

== system tqd/TQD/Input_Convert/Input Signal Convert/Big Mike Combo V2 /Combo Key Detection/Function3/Key3/Maintain ==
  Input : Inport
  Action Port : ActionPort
  KeepKey3 : Outport
  wires:
  Input/1 -> KeepKey3/1

== system tqd/TQD/Input_Convert/Input Signal Convert/Big Mike Combo V2 /Combo Key Detection/Function3/Key3/Reset ==
  Action Port : ActionPort
  Constant : Constant  Value=ENUM_COMBOKEY_NONE
  ResetToZero : Outport
  wires:
  Constant/1 -> ResetToZero/1

== system tqd/TQD/Input_Convert/Input Signal Convert/Big Mike Combo V2 /Combo Key Detection/Function3/Key3/Write ==
  Input : Inport
  Action Port : ActionPort
  WriteCMD : Outport
  wires:
  Input/1 -> WriteCMD/1

== system tqd/TQD/Input_Convert/Input Signal Convert/Big Mike Combo V2 /Combo Key Detection/Function3/Key4/Maintain ==
  Input : Inport
  Action Port : ActionPort
  KeepKey4 : Outport
  wires:
  Input/1 -> KeepKey4/1

== system tqd/TQD/Input_Convert/Input Signal Convert/Big Mike Combo V2 /Combo Key Detection/Function3/Key4/Reset ==
  Action Port : ActionPort
  Constant : Constant  Value=ENUM_COMBOKEY_NONE
  ResetToZero : Outport
  wires:
  Constant/1 -> ResetToZero/1

== system tqd/TQD/Input_Convert/Input Signal Convert/Big Mike Combo V2 /Combo Key Detection/Function3/Key4/Write ==
  Input : Inport
  Action Port : ActionPort
  WriteCMD : Outport
  wires:
  Input/1 -> WriteCMD/1

== system tqd/TQD/Input_Convert/Input Signal Convert/Big Mike Combo V2 /Combo Key Detection/Function3/Key5/Maintain ==
  Input : Inport
  Action Port : ActionPort
  KeepKey5 : Outport
  wires:
  Input/1 -> KeepKey5/1

== system tqd/TQD/Input_Convert/Input Signal Convert/Big Mike Combo V2 /Combo Key Detection/Function3/Key5/Reset ==
  Action Port : ActionPort
  Constant : Constant  Value=ENUM_COMBOKEY_NONE
  ResetToZero : Outport
  wires:
  Constant/1 -> ResetToZero/1

== system tqd/TQD/Input_Convert/Input Signal Convert/Big Mike Combo V2 /Combo Key Detection/Function3/Key5/Write ==
  Input : Inport
  Action Port : ActionPort
  WriteCMD : Outport
  wires:
  Input/1 -> WriteCMD/1

== system tqd/TQD/Input_Convert/Input Signal Convert/Big Mike Combo V2 /Combo Key Detection/Function3/Key6/Maintain ==
  Input : Inport
  Action Port : ActionPort
  KeepKey6 : Outport
  wires:
  Input/1 -> KeepKey6/1

== system tqd/TQD/Input_Convert/Input Signal Convert/Big Mike Combo V2 /Combo Key Detection/Function3/Key6/Reset ==
  Action Port : ActionPort
  Constant : Constant  Value=ENUM_COMBOKEY_NONE
  ResetToZero : Outport
  wires:
  Constant/1 -> ResetToZero/1

== system tqd/TQD/Input_Convert/Input Signal Convert/Big Mike Combo V2 /Combo Key Detection/Function3/Key6/Write ==
  Input : Inport
  Action Port : ActionPort
  WriteCMD : Outport
  wires:
  Input/1 -> WriteCMD/1

== system tqd/TQD/Input_Convert/Input Signal Convert/Big Mike Combo V2 /Combo Key Detection/Function3/Key7/Maintain ==
  Input : Inport
  Action Port : ActionPort
  KeepKey7 : Outport
  wires:
  Input/1 -> KeepKey7/1

== system tqd/TQD/Input_Convert/Input Signal Convert/Big Mike Combo V2 /Combo Key Detection/Function3/Key7/Reset ==
  Action Port : ActionPort
  Constant : Constant  Value=ENUM_COMBOKEY_NONE
  ResetToZero : Outport
  wires:
  Constant/1 -> ResetToZero/1

== system tqd/TQD/Input_Convert/Input Signal Convert/Big Mike Combo V2 /Combo Key Detection/Function3/Key7/Write ==
  Input : Inport
  Action Port : ActionPort
  WriteCMD : Outport
  wires:
  Input/1 -> WriteCMD/1

== system tqd/TQD/Input_Convert/Input Signal Convert/Big Mike Combo V2 /Combo Key Detection/Function3/Key8/Maintain ==
  Input : Inport
  Action Port : ActionPort
  KeepKey8 : Outport
  wires:
  Input/1 -> KeepKey8/1

== system tqd/TQD/Input_Convert/Input Signal Convert/Big Mike Combo V2 /Combo Key Detection/Function3/Key8/Reset ==
  Action Port : ActionPort
  Constant : Constant  Value=ENUM_COMBOKEY_NONE
  ResetToZero : Outport
  wires:
  Constant/1 -> ResetToZero/1

== system tqd/TQD/Input_Convert/Input Signal Convert/Big Mike Combo V2 /Combo Key Detection/Function3/Key8/Write ==
  Input : Inport
  Action Port : ActionPort
  WriteCMD : Outport
  wires:
  Input/1 -> WriteCMD/1

== system tqd/TQD/Input_Convert/Input Signal Convert/Big Mike Combo V2 /Combo Key Detection/Function4 /Key1/Maintain ==
  Input : Inport
  Action Port : ActionPort
  KeepKey1 : Outport
  wires:
  Input/1 -> KeepKey1/1

== system tqd/TQD/Input_Convert/Input Signal Convert/Big Mike Combo V2 /Combo Key Detection/Function4 /Key1/Reset ==
  Action Port : ActionPort
  Constant : Constant  Value=ENUM_COMBOKEY_NONE
  ResetToZero : Outport
  wires:
  Constant/1 -> ResetToZero/1

== system tqd/TQD/Input_Convert/Input Signal Convert/Big Mike Combo V2 /Combo Key Detection/Function4 /Key1/Write ==
  Input : Inport
  Action Port : ActionPort
  WriteCMD : Outport
  wires:
  Input/1 -> WriteCMD/1

== system tqd/TQD/Input_Convert/Input Signal Convert/Big Mike Combo V2 /Combo Key Detection/Function4 /Key2/Maintain ==
  Input : Inport
  Action Port : ActionPort
  KeepKey2 : Outport
  wires:
  Input/1 -> KeepKey2/1

== system tqd/TQD/Input_Convert/Input Signal Convert/Big Mike Combo V2 /Combo Key Detection/Function4 /Key2/Reset ==
  Action Port : ActionPort
  Constant : Constant  Value=ENUM_COMBOKEY_NONE
  ResetToZero : Outport
  wires:
  Constant/1 -> ResetToZero/1

== system tqd/TQD/Input_Convert/Input Signal Convert/Big Mike Combo V2 /Combo Key Detection/Function4 /Key2/Write ==
  Input : Inport
  Action Port : ActionPort
  WriteCMD : Outport
  wires:
  Input/1 -> WriteCMD/1

== system tqd/TQD/Input_Convert/Input Signal Convert/Big Mike Combo V2 /Combo Key Detection/Function4 /Key3/Maintain ==
  Input : Inport
  Action Port : ActionPort
  KeepKey3 : Outport
  wires:
  Input/1 -> KeepKey3/1

== system tqd/TQD/Input_Convert/Input Signal Convert/Big Mike Combo V2 /Combo Key Detection/Function4 /Key3/Reset ==
  Action Port : ActionPort
  Constant : Constant  Value=ENUM_COMBOKEY_NONE
  ResetToZero : Outport
  wires:
  Constant/1 -> ResetToZero/1

== system tqd/TQD/Input_Convert/Input Signal Convert/Big Mike Combo V2 /Combo Key Detection/Function4 /Key3/Write ==
  Input : Inport
  Action Port : ActionPort
  WriteCMD : Outport
  wires:
  Input/1 -> WriteCMD/1

== system tqd/TQD/Input_Convert/Input Signal Convert/Big Mike Combo V2 /Combo Key Detection/Function4 /Key4/Maintain ==
  Input : Inport
  Action Port : ActionPort
  KeepKey4 : Outport
  wires:
  Input/1 -> KeepKey4/1

== system tqd/TQD/Input_Convert/Input Signal Convert/Big Mike Combo V2 /Combo Key Detection/Function4 /Key4/Reset ==
  Action Port : ActionPort
  Constant : Constant  Value=ENUM_COMBOKEY_NONE
  ResetToZero : Outport
  wires:
  Constant/1 -> ResetToZero/1

== system tqd/TQD/Input_Convert/Input Signal Convert/Big Mike Combo V2 /Combo Key Detection/Function4 /Key4/Write ==
  Input : Inport
  Action Port : ActionPort
  WriteCMD : Outport
  wires:
  Input/1 -> WriteCMD/1

== system tqd/TQD/Input_Convert/Input Signal Convert/Big Mike Combo V2 /Combo Key Detection/Function4 /Key5/Maintain ==
  Input : Inport
  Action Port : ActionPort
  KeepKey5 : Outport
  wires:
  Input/1 -> KeepKey5/1

== system tqd/TQD/Input_Convert/Input Signal Convert/Big Mike Combo V2 /Combo Key Detection/Function4 /Key5/Reset ==
  Action Port : ActionPort
  Constant : Constant  Value=ENUM_COMBOKEY_NONE
  ResetToZero : Outport
  wires:
  Constant/1 -> ResetToZero/1

== system tqd/TQD/Input_Convert/Input Signal Convert/Big Mike Combo V2 /Combo Key Detection/Function4 /Key5/Write ==
  Input : Inport
  Action Port : ActionPort
  WriteCMD : Outport
  wires:
  Input/1 -> WriteCMD/1

== system tqd/TQD/Input_Convert/Input Signal Convert/Big Mike Combo V2 /Combo Key Detection/Function4 /Key6/Maintain ==
  Input : Inport
  Action Port : ActionPort
  KeepKey6 : Outport
  wires:
  Input/1 -> KeepKey6/1

== system tqd/TQD/Input_Convert/Input Signal Convert/Big Mike Combo V2 /Combo Key Detection/Function4 /Key6/Reset ==
  Action Port : ActionPort
  Constant : Constant  Value=ENUM_COMBOKEY_NONE
  ResetToZero : Outport
  wires:
  Constant/1 -> ResetToZero/1

== system tqd/TQD/Input_Convert/Input Signal Convert/Big Mike Combo V2 /Combo Key Detection/Function4 /Key6/Write ==
  Input : Inport
  Action Port : ActionPort
  WriteCMD : Outport
  wires:
  Input/1 -> WriteCMD/1

== system tqd/TQD/Input_Convert/Input Signal Convert/Big Mike Combo V2 /Combo Key Detection/Function4 /Key7/Maintain ==
  Input : Inport
  Action Port : ActionPort
  KeepKey7 : Outport
  wires:
  Input/1 -> KeepKey7/1

== system tqd/TQD/Input_Convert/Input Signal Convert/Big Mike Combo V2 /Combo Key Detection/Function4 /Key7/Reset ==
  Action Port : ActionPort
  Constant : Constant  Value=ENUM_COMBOKEY_NONE
  ResetToZero : Outport
  wires:
  Constant/1 -> ResetToZero/1

== system tqd/TQD/Input_Convert/Input Signal Convert/Big Mike Combo V2 /Combo Key Detection/Function4 /Key7/Write ==
  Input : Inport
  Action Port : ActionPort
  WriteCMD : Outport
  wires:
  Input/1 -> WriteCMD/1

== system tqd/TQD/Input_Convert/Input Signal Convert/Big Mike Combo V2 /Combo Key Detection/Function4 /Key8/Maintain ==
  Input : Inport
  Action Port : ActionPort
  KeepKey8 : Outport
  wires:
  Input/1 -> KeepKey8/1

== system tqd/TQD/Input_Convert/Input Signal Convert/Big Mike Combo V2 /Combo Key Detection/Function4 /Key8/Reset ==
  Action Port : ActionPort
  Constant : Constant  Value=ENUM_COMBOKEY_NONE
  ResetToZero : Outport
  wires:
  Constant/1 -> ResetToZero/1

== system tqd/TQD/Input_Convert/Input Signal Convert/Big Mike Combo V2 /Combo Key Detection/Function4 /Key8/Write ==
  Input : Inport
  Action Port : ActionPort
  WriteCMD : Outport
  wires:
  Input/1 -> WriteCMD/1

== system tqd/TQD/Input_Convert/Input Signal Convert/Big Mike Combo V2 /Combo Key Detection/Function5/Key1/Maintain ==
  Input : Inport
  Action Port : ActionPort
  KeepKey1 : Outport
  wires:
  Input/1 -> KeepKey1/1

== system tqd/TQD/Input_Convert/Input Signal Convert/Big Mike Combo V2 /Combo Key Detection/Function5/Key1/Reset ==
  Action Port : ActionPort
  Constant : Constant  Value=ENUM_COMBOKEY_NONE
  ResetToZero : Outport
  wires:
  Constant/1 -> ResetToZero/1

== system tqd/TQD/Input_Convert/Input Signal Convert/Big Mike Combo V2 /Combo Key Detection/Function5/Key1/Write ==
  Input : Inport
  Action Port : ActionPort
  WriteCMD : Outport
  wires:
  Input/1 -> WriteCMD/1

== system tqd/TQD/Input_Convert/Input Signal Convert/Big Mike Combo V2 /Combo Key Detection/Function5/Key2/Maintain ==
  Input : Inport
  Action Port : ActionPort
  KeepKey2 : Outport
  wires:
  Input/1 -> KeepKey2/1

== system tqd/TQD/Input_Convert/Input Signal Convert/Big Mike Combo V2 /Combo Key Detection/Function5/Key2/Reset ==
  Action Port : ActionPort
  Constant : Constant  Value=ENUM_COMBOKEY_NONE
  ResetToZero : Outport
  wires:
  Constant/1 -> ResetToZero/1

== system tqd/TQD/Input_Convert/Input Signal Convert/Big Mike Combo V2 /Combo Key Detection/Function5/Key2/Write ==
  Input : Inport
  Action Port : ActionPort
  WriteCMD : Outport
  wires:
  Input/1 -> WriteCMD/1

== system tqd/TQD/Input_Convert/Input Signal Convert/Big Mike Combo V2 /Combo Key Detection/Function5/Key3/Maintain ==
  Input : Inport
  Action Port : ActionPort
  KeepKey3 : Outport
  wires:
  Input/1 -> KeepKey3/1

== system tqd/TQD/Input_Convert/Input Signal Convert/Big Mike Combo V2 /Combo Key Detection/Function5/Key3/Reset ==
  Action Port : ActionPort
  Constant : Constant  Value=ENUM_COMBOKEY_NONE
  ResetToZero : Outport
  wires:
  Constant/1 -> ResetToZero/1

== system tqd/TQD/Input_Convert/Input Signal Convert/Big Mike Combo V2 /Combo Key Detection/Function5/Key3/Write ==
  Input : Inport
  Action Port : ActionPort
  WriteCMD : Outport
  wires:
  Input/1 -> WriteCMD/1

== system tqd/TQD/Input_Convert/Input Signal Convert/Big Mike Combo V2 /Combo Key Detection/Function5/Key4/Maintain ==
  Input : Inport
  Action Port : ActionPort
  KeepKey4 : Outport
  wires:
  Input/1 -> KeepKey4/1

== system tqd/TQD/Input_Convert/Input Signal Convert/Big Mike Combo V2 /Combo Key Detection/Function5/Key4/Reset ==
  Action Port : ActionPort
  Constant : Constant  Value=ENUM_COMBOKEY_NONE
  ResetToZero : Outport
  wires:
  Constant/1 -> ResetToZero/1

== system tqd/TQD/Input_Convert/Input Signal Convert/Big Mike Combo V2 /Combo Key Detection/Function5/Key4/Write ==
  Input : Inport
  Action Port : ActionPort
  WriteCMD : Outport
  wires:
  Input/1 -> WriteCMD/1

== system tqd/TQD/Input_Convert/Input Signal Convert/Big Mike Combo V2 /Combo Key Detection/Function5/Key5/Maintain ==
  Input : Inport
  Action Port : ActionPort
  KeepKey5 : Outport
  wires:
  Input/1 -> KeepKey5/1

== system tqd/TQD/Input_Convert/Input Signal Convert/Big Mike Combo V2 /Combo Key Detection/Function5/Key5/Reset ==
  Action Port : ActionPort
  Constant : Constant  Value=ENUM_COMBOKEY_NONE
  ResetToZero : Outport
  wires:
  Constant/1 -> ResetToZero/1

== system tqd/TQD/Input_Convert/Input Signal Convert/Big Mike Combo V2 /Combo Key Detection/Function5/Key5/Write ==
  Input : Inport
  Action Port : ActionPort
  WriteCMD : Outport
  wires:
  Input/1 -> WriteCMD/1

== system tqd/TQD/Input_Convert/Input Signal Convert/Big Mike Combo V2 /Combo Key Detection/Function5/Key6/Maintain ==
  Input : Inport
  Action Port : ActionPort
  KeepKey6 : Outport
  wires:
  Input/1 -> KeepKey6/1

== system tqd/TQD/Input_Convert/Input Signal Convert/Big Mike Combo V2 /Combo Key Detection/Function5/Key6/Reset ==
  Action Port : ActionPort
  Constant : Constant  Value=ENUM_COMBOKEY_NONE
  ResetToZero : Outport
  wires:
  Constant/1 -> ResetToZero/1

== system tqd/TQD/Input_Convert/Input Signal Convert/Big Mike Combo V2 /Combo Key Detection/Function5/Key6/Write ==
  Input : Inport
  Action Port : ActionPort
  WriteCMD : Outport
  wires:
  Input/1 -> WriteCMD/1

== system tqd/TQD/Input_Convert/Input Signal Convert/Big Mike Combo V2 /Combo Key Detection/Function5/Key7/Maintain ==
  Input : Inport
  Action Port : ActionPort
  KeepKey7 : Outport
  wires:
  Input/1 -> KeepKey7/1

== system tqd/TQD/Input_Convert/Input Signal Convert/Big Mike Combo V2 /Combo Key Detection/Function5/Key7/Reset ==
  Action Port : ActionPort
  Constant : Constant  Value=ENUM_COMBOKEY_NONE
  ResetToZero : Outport
  wires:
  Constant/1 -> ResetToZero/1

== system tqd/TQD/Input_Convert/Input Signal Convert/Big Mike Combo V2 /Combo Key Detection/Function5/Key7/Write ==
  Input : Inport
  Action Port : ActionPort
  WriteCMD : Outport
  wires:
  Input/1 -> WriteCMD/1

== system tqd/TQD/Input_Convert/Input Signal Convert/Big Mike Combo V2 /Combo Key Detection/Function5/Key8/Maintain ==
  Input : Inport
  Action Port : ActionPort
  KeepKey8 : Outport
  wires:
  Input/1 -> KeepKey8/1

== system tqd/TQD/Input_Convert/Input Signal Convert/Big Mike Combo V2 /Combo Key Detection/Function5/Key8/Reset ==
  Action Port : ActionPort
  Constant : Constant  Value=ENUM_COMBOKEY_NONE
  ResetToZero : Outport
  wires:
  Constant/1 -> ResetToZero/1

== system tqd/TQD/Input_Convert/Input Signal Convert/Big Mike Combo V2 /Combo Key Detection/Function5/Key8/Write ==
  Input : Inport
  Action Port : ActionPort
  WriteCMD : Outport
  wires:
  Input/1 -> WriteCMD/1

== stateflow chart tqd/TQD/Input_Convert/Input Signal Convert/Engineering Mode Disable Flasher/Chart ==
  state init
    en:
    time_cnt = ZERO_INT;
    ON_flg = TRUE;
    OFF_flg = FALSE;
    out = FALSE;
    CycleCnt_cnt = FALSE;
  state OFF
    en:
    out = FALSE;
    time_cnt = ZERO_INT;
    OFF -> (junction 38) [order 1]
    (junction 38) -> OFF : {time_cnt = time_cnt + ZERO_INT;}
  state ON
    en:
    out = TRUE;
    time_cnt = ZERO_INT;
    du:
    time_cnt = time_cnt + ONE_INT;
  state WAIT
    en:
    out = FALSE;
    time_cnt = ZERO_INT;
    du:
    time_cnt = time_cnt + ONE_INT;
  (default) -> init
  init -> (junction 57)
  (junction 57) -> ON : [ON_flg && VSCP_FlasherEn_flg]
  OFF -> (junction 46) [order 2] : [time_cnt > OFF_cnt]
  (junction 46) -> (junction 47) : {time_cnt = ZERO_INT;
      |  ON_flg = TRUE;
      |  OFF_flg = FALSE;
      |  CycleCnt_cnt = CycleCnt_cnt +ONE_INT;}
  (junction 47) -> ON : [ON_flg]
  ON -> (junction 44) : [time_cnt > ON_cnt]
  (junction 44) -> (junction 42) : {time_cnt = ZERO_INT;
      |  ON_flg = FALSE;
      |  OFF_flg = TRUE;}
  (junction 42) -> OFF : [OFF_flg]
  OFF -> (junction 66) [order 1] : [time_cnt > OFF_cnt && CycleCnt_cnt >= Cycle_cnt]
  (junction 66) -> WAIT : {time_cnt = ZERO_INT;}
  (junction 62) -> ON : {time_cnt = ZERO_INT;
      |  ON_flg = TRUE;
      |  OFF_flg = FALSE;
      |  CycleCnt_cnt = ZERO_INT;}
  WAIT -> (junction 62) : [time_cnt >= WAIT_cnt && VSCP_FlasherEn_flg]
  data: ON_cnt input; OFF_cnt input; WAIT_cnt input; Cycle_cnt input; out output boolean; time_cnt local uint8; OFF_flg local boolean; ON_flg local boolean; CycleCnt_cnt local uint8; VSCP_FlasherEn_flg input; FALSE parameter; TRUE parameter; ONE_INT parameter; ZERO_INT parameter

== stateflow chart tqd/TQD/Main/Torque Coordination/Coordination Machine ==
  (default) -> (junction 1)
  (junction 1) -> (junction 8) [order 1] : [VTQD_NoSuitbleGear_flg]
  (junction 1) -> (junction 12) [order 2] : {
      | VTQD_CoordTqDem_Nm = VTQD_DriverTqDem_Nm;
      | }
  (junction 8) -> (junction 10) : {
      | VTQD_CoordTqDem_Nm = KTQD_MotoringTqDemN_Nm;
      | }
  data: VTQD_NoSuitbleGear_flg input; KTQD_MotoringTqDemN_Nm parameter; VTQD_DriverTqDem_Nm input; VTQD_CoordTqDem_Nm output
